simulink model "x8_ind_midpoint_with_compensation"  (R2024b)
settings: Solver=VariableStepAuto  StartTime=0.0  StopTime=1  RelTol=1e-3
libraries: spsRMSLib x10, spsVoltageMeasurementLib x9, spsSeriesRLCBranchLib x8, spsACVoltageSourceLib x5, spsCurrentMeasurementLib x1, sps_lib x1
settings Model: Creator=N I T R O  LastModifiedBy=N I T R O
settings DataIOCC: ReturnWorkspaceOutputs=off

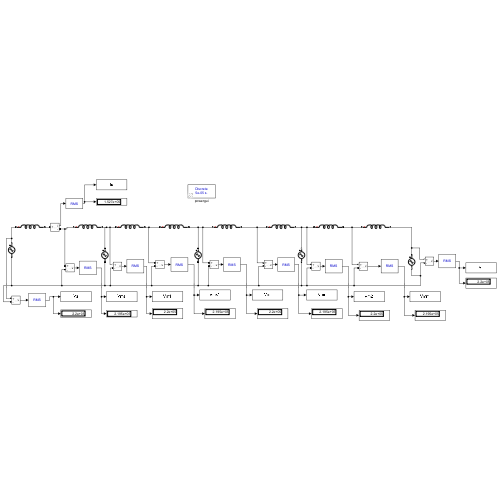
[thumbnail: Simulink's stored preview of the top-level diagram]
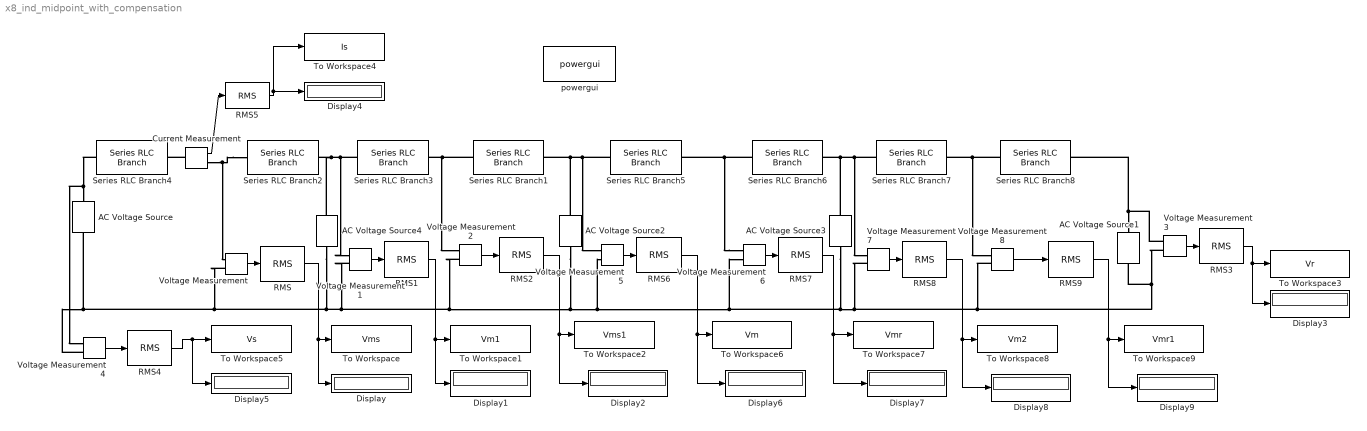
== system x8_ind_midpoint_with_compensation ==
  AC Voltage Source : spsACVoltageSourceLib/AC Voltage Source  Amplitude=220e3*sqrt(2)  Phase=15  Frequency=50  SampleTime=0  Measurements=None  BusType=swing  Pref=10e3  Qref=0  Qmin=-inf  Qmax=+inf
  AC Voltage Source1 : spsACVoltageSourceLib/AC Voltage Source  Amplitude=220e3*sqrt(2)  Phase=-15  Frequency=50  SampleTime=0  Measurements=None  BusType=swing  Pref=10e3  Qref=0  Qmin=-inf  Qmax=+inf
  AC Voltage Source2 : spsACVoltageSourceLib/AC Voltage Source  Amplitude=220e3*sqrt(2)  Phase=0  Frequency=50  SampleTime=0  Measurements=None  BusType=swing  Pref=10e3  Qref=0  Qmin=-inf  Qmax=+inf
  AC Voltage Source3 : spsACVoltageSourceLib/AC Voltage Source  Amplitude=220e3*sqrt(2)  Phase=-15/2  Frequency=50  SampleTime=0  Measurements=None  BusType=swing  Pref=10e3  Qref=0  Qmin=-inf  Qmax=+inf
  AC Voltage Source4 : spsACVoltageSourceLib/AC Voltage Source  Amplitude=220e3*sqrt(2)  Phase=15/2  Frequency=50  SampleTime=0  Measurements=None  BusType=swing  Pref=10e3  Qref=0  Qmin=-inf  Qmax=+inf
  Current Measurement : spsCurrentMeasurementLib/Current Measurement  PhasorSimulation=off  OutputType=Complex  PSBequivalent=0
  Display{,1..9} (10 alike) : Display
  RMS{,1..9} (10 alike) : spsRMSLib/RMS  TrueRMS=on  Freq=50  RMSInit=120  Ts=0
  Series RLC Branch{1..8} (8 alike) : spsSeriesRLCBranchLib/Series RLC Branch  LConnTagsString=__new0  RConnTagsString=__new0  BranchType=L  Resistance=1  Inductance=1.2e-3/4  SetiL0=off  InitialCurrent=0  Capacitance=1e-6  Setx0=off  InitialVoltage=0  Measurements=None
  To Workspace : ToWorkspace  VariableName=Vms  SampleTime=-1
  To Workspace1 : ToWorkspace  VariableName=Vm1  SampleTime=-1
  To Workspace2 : ToWorkspace  VariableName=Vms1  SampleTime=-1
  To Workspace3 : ToWorkspace  VariableName=Vr  SampleTime=-1
  To Workspace4 : ToWorkspace  VariableName=Is  SampleTime=-1
  To Workspace5 : ToWorkspace  VariableName=Vs  SampleTime=-1
  To Workspace6 : ToWorkspace  VariableName=Vm  SampleTime=-1
  To Workspace7 : ToWorkspace  VariableName=Vmr  SampleTime=-1
  To Workspace8 : ToWorkspace  VariableName=Vm2  SampleTime=-1
  To Workspace9 : ToWorkspace  VariableName=Vmr1  SampleTime=-1
  Voltage Measurement{,1..8} (9 alike) : spsVoltageMeasurementLib/Voltage Measurement  PhasorSimulation=off  OutputType=Complex  PSBequivalent=0
  powergui : sps_lib/powergui  Priority=1  SimulationMode=Discrete  SampleTime=5e-05  frequency=60  Iterations=50  frequencyindice=50  Pbase=100e6  ErrMax=1e-4  UnitsV=kV  UnitsW=MW  buscounter=0  FunctionMessages=off  echomessages=off  EnableUseOfTLC=off  CurrentSourceSwitches=off  DisableSnubberDevices=off  DisableRonSwitches=off  DisableVfSwitches=off  DisplayEquations=off  AutomaticDiscreteSolvers=off  SolverType=Tustin/Backward Euler (TBE)  Interpol=off  ExternalGateDelay=off  methode=off  Ts=100  x0status=blocks  SPID=on  SwTol=0  HookPort=off  NonlinearTolerance=1e-4  nMaxIteration=100  ContinueOnMaxIteration=off  RestoreLinks=warning  ResistiveCurrentMeasurement=off  Frange=[0:2:500]  Ylog=off  Xlog=on  ShowGrid=off  save=off  variable=ZData  structure=0  ZoomFFT=off  StartTime=0.0  cycles=1  DisplayStyle=1  fundamental=60  FreqAxis=off  MaxFrequency=1000  frequencyindicesteady=1  RmsSteady=1  display=off
  wires:
  Voltage Measurement/1 -> RMS/1
  RMS4/1 -> Display5/1, To Workspace5/1
  Voltage Measurement4/1 -> RMS4/1
  RMS2/1 -> Display2/1, To Workspace2/1
  Voltage Measurement1/1 -> RMS1/1
  RMS3/1 -> Display3/1, To Workspace3/1
  RMS1/1 -> Display1/1, To Workspace1/1
  Voltage Measurement2/1 -> RMS2/1
  Voltage Measurement3/1 -> RMS3/1
  RMS5/1 -> To Workspace4/1, Display4/1
  Current Measurement/1 -> RMS5/1
  RMS/1 -> Display/1, To Workspace/1
  Voltage Measurement5/1 -> RMS6/1
  RMS6/1 -> To Workspace6/1, Display6/1
  RMS7/1 -> To Workspace7/1, Display7/1
  Voltage Measurement6/1 -> RMS7/1
  Voltage Measurement7/1 -> RMS8/1
  RMS8/1 -> To Workspace8/1, Display8/1
  RMS9/1 -> Display9/1, To Workspace9/1
  Voltage Measurement8/1 -> RMS9/1
  connections:
  Voltage Measurement3/LConn2 -- Voltage Measurement8/LConn2 -- AC Voltage Source3/LConn1 -- AC Voltage Source2/LConn1 -- Voltage Measurement2/LConn2 -- Voltage Measurement1/LConn2 -- AC Voltage Source4/LConn1 -- Voltage Measurement/LConn2 -- Voltage Measurement4/LConn2 -- AC Voltage Source/LConn1 -- Voltage Measurement5/LConn2 -- Voltage Measurement6/LConn2 -- Voltage Measurement7/LConn2 -- AC Voltage Source1/LConn1
  AC Voltage Source/RConn1 -- Series RLC Branch4/LConn1 -- Voltage Measurement4/LConn1
  Voltage Measurement1/LConn1 -- Series RLC Branch3/LConn1 -- AC Voltage Source4/RConn1 -- Series RLC Branch2/RConn1
  Series RLC Branch2/LConn1 -- Current Measurement/RConn1 -- Voltage Measurement/LConn1
  Series RLC Branch3/RConn1 -- Series RLC Branch1/LConn1 -- Voltage Measurement2/LConn1
  Current Measurement/LConn1 -- Series RLC Branch4/RConn1
  Series RLC Branch5/LConn1 -- AC Voltage Source2/RConn1 -- Series RLC Branch1/RConn1 -- Voltage Measurement5/LConn1
  Voltage Measurement6/LConn1 -- Series RLC Branch6/LConn1 -- Series RLC Branch5/RConn1
  Series RLC Branch7/LConn1 -- AC Voltage Source3/RConn1 -- Series RLC Branch6/RConn1 -- Voltage Measurement7/LConn1
  Series RLC Branch8/LConn1 -- Voltage Measurement8/LConn1 -- Series RLC Branch7/RConn1
  Voltage Measurement3/LConn1 -- Series RLC Branch8/RConn1 -- AC Voltage Source1/RConn1
